simulink model "GFF"  (R2024b)
settings: Solver=VariableStepAuto  StartTime=0.0  StopTime=10.0  RelTol=1e-3
settings Model: Creator=Ilya  LastModifiedBy=Ilya

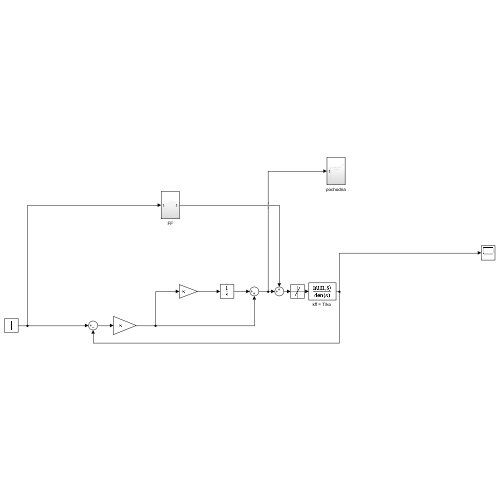
[thumbnail: Simulink's stored preview of the top-level diagram]
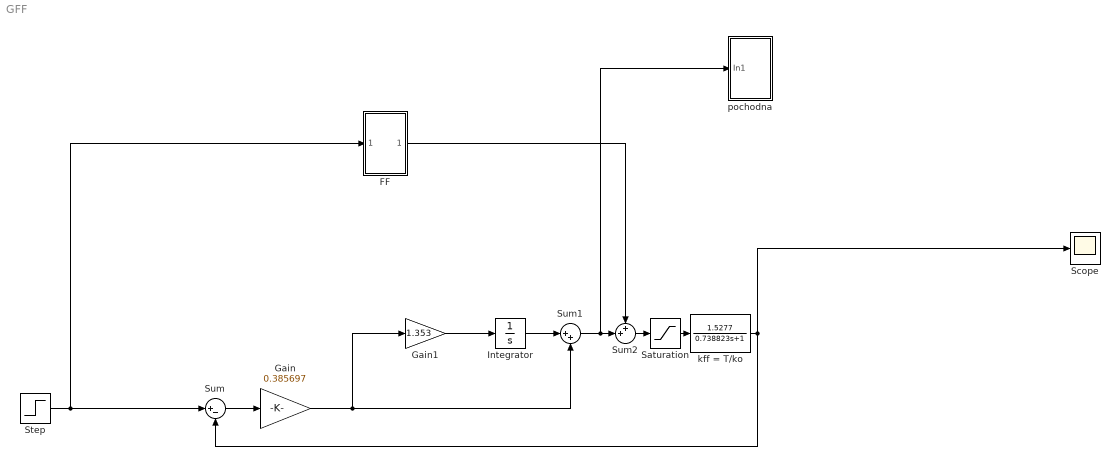
== system GFF ==
  FF : Subsystem
  Gain : Gain  Gain=0.385697
  Gain1 : Gain  Gain=1.353
  Integrator : Integrator
  Saturation : Saturate  UpperLimit=1000  LowerLimit=0
  Scope : Scope
  Step : Step  Time=0  After=100  SampleTime=0
  Sum : Sum  Inputs=|+-
  Sum1 : Sum  Inputs=|++
  Sum2 : Sum  Inputs=++|
  "kff = T/ko " : TransferFcn  Numerator=[1.5277]  Denominator=[0.738823 1]
  pochodna : Subsystem
  wires:
  FF/1(Out1) -> Sum2/1
  Sum1/1 -> pochodna/1(In1), Sum2/2
  Sum2/1 -> Saturation/1
  Step/1 -> FF/1(In1), Sum/1
  Gain1/1 -> Integrator/1
  "kff = T/ko "/1 -> Scope/1, Sum/2
  Gain/1 -> Gain1/1, Sum1/2
  Integrator/1 -> Sum1/1
  Saturation/1 -> "kff = T/ko "/1
  Sum/1 -> Gain/1

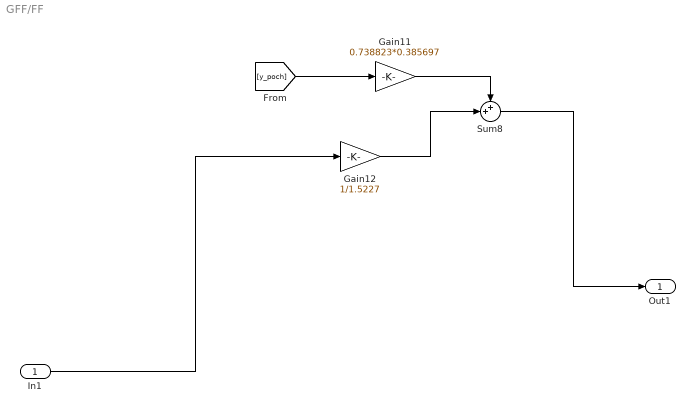
== system GFF/FF ==
  In1 : Inport
  Gain11 : Gain  Gain=0.738823*0.385697
  Gain12 : Gain  Gain=1/1.5227
  Sum8 : Sum  Inputs=++|
  Out1 : Outport
  wires:
  Gain12/1 -> Sum8/2
  [y_poch] -> Gain11/1
  Gain11/1 -> Sum8/1
  In1/1 -> Gain12/1
  Sum8/1 -> Out1/1

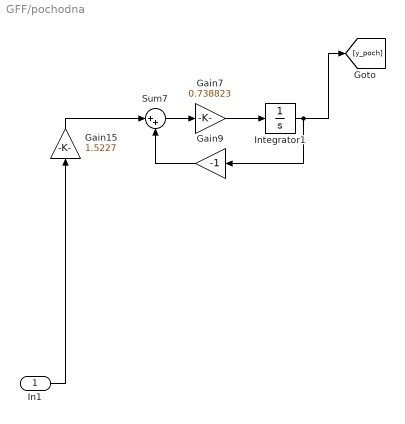
== system GFF/pochodna ==
  In1 : Inport
  Gain15 : Gain  Gain=1.5227
  Gain7 : Gain  Gain=0.738823
  Gain9 : Gain  Gain=-1
  Integrator1 : Integrator
  Sum7 : Sum  Inputs=|++
  wires:
  Gain15/1 -> Sum7/1
  Integrator1/1 -> Gain9/1, [y_poch]
  Gain9/1 -> Sum7/2
  Gain7/1 -> Integrator1/1
  In1/1 -> Gain15/1
  Sum7/1 -> Gain7/1
